simulink library "environment_lib"  (R2016b)
settings: Solver=ode45  StartTime=0.0  StopTime=10.0  RelTol=1e-3  EnableMultiTasking=on
undefined symbols (not defined in the file or in its folder): DT_aero, DT_grav, DT_solar, env_acc_eci, fsw_params, init_pos_eci, init_vel_eci, mag_vector_eci, MD_SC_resdipole, sun_vec_eci
libraries: time_conversion_lib x2, bus_stubs_template x2, GPS_time_lib x1, coord_rotation_lib x1, disturbances_lib x1, tle2eci_coarse_lib x1
settings Model: Creator=bbarz_000  LastModifiedBy=evich
settings DataIOCC: LimitDataPoints=on
settings OptimizationCC: LifeSpan=inf
settings DebuggingCC: AllowSymbolicDim=off  SFUnexpectedBacktrackingDiag=warning  SFNoUnconditionalDefaultTransitionDiag=warning  SFExecutionAtInitializationDiag=none
settings GRTTargetCC: TargetLangStandard=C89/C90 (ANSI)  GeneratePreprocessorConditionals=Disable all
settings ConfigComp: CovMetricSettings=dw  CovHtmlReporting=on  CovSaveCumulativeToWorkspaceVar=on  CovSaveSingleToWorkspaceVar=on  CovExternalEMLEnable=off

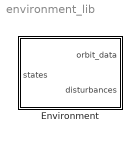
== system environment_lib ==
  Environment : Subsystem

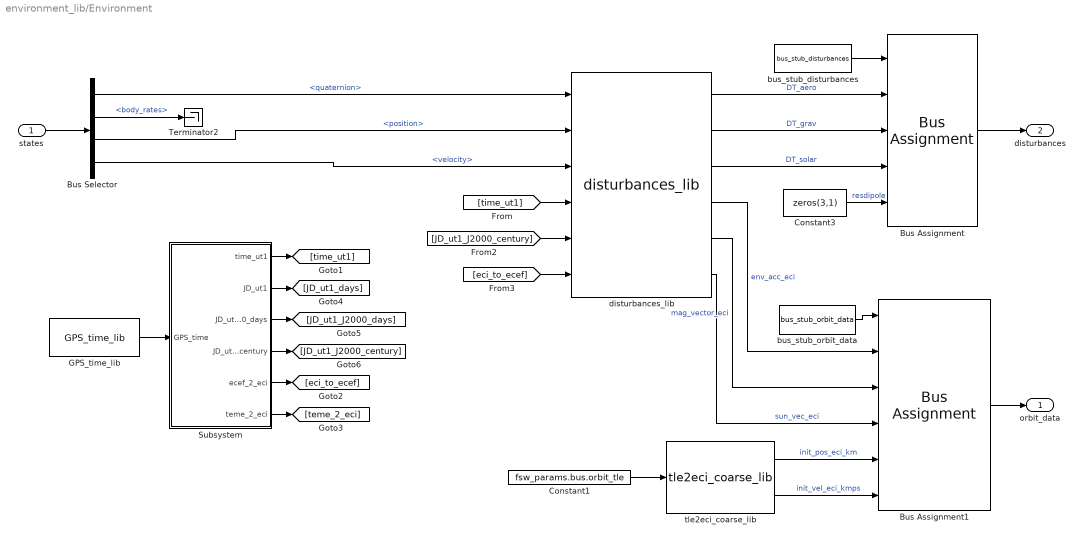
== system environment_lib/Environment ==
  states : Inport  OutDataTypeStr=Bus: states
  Bus Assignment : BusAssignment  AssignedSignals=DT_aero,DT_grav,DT_solar,MD_SC_resdipole
  Bus Assignment1 : BusAssignment  AssignedSignals=env_acc_eci,mag_vector_eci,sun_vec_eci,init_pos_eci,init_vel_eci
  Bus Selector : BusSelector  OutputSignals=quaternion,body_rates,position,velocity
  Constant1 : Constant  Value=fsw_params.bus.orbit_tle
  Constant3 : Constant  Value=zeros(3,1)
  GPS_time_lib : GPS_time_lib/GPS_time_lib
  Subsystem : Subsystem
  Terminator2 : Terminator
  bus_stub_disturbances : bus_stubs_template/bus_stub_disturbances
  bus_stub_orbit_data : bus_stubs_template/bus_stub_orbit_data
  disturbances_lib : disturbances_lib/disturbances_lib
  tle2eci_coarse_lib : tle2eci_coarse_lib/tle2eci_coarse_lib
  orbit_data : Outport
  disturbances : Outport  Port=2
  wires:
  tle2eci_coarse_lib/2 -> Bus Assignment1/6  "init_vel_eci_kmps"
  tle2eci_coarse_lib/1 -> Bus Assignment1/5  "init_pos_eci_km"
  Constant1/1 -> tle2eci_coarse_lib/1
  bus_stub_disturbances/1 -> Bus Assignment/1
  Bus Assignment/1 -> disturbances/1
  states/1 -> Bus Selector/1
  Bus Selector/1 -> disturbances_lib/1  "<quaternion>"
  Bus Selector/2 -> Terminator2/1  "<body_rates>"
  Bus Selector/3 -> disturbances_lib/2  "<position>"
  Bus Selector/4 -> disturbances_lib/3  "<velocity>"
  [time_ut1] -> disturbances_lib/4
  Constant3/1 -> Bus Assignment/5  "resdipole"
  bus_stub_orbit_data/1 -> Bus Assignment1/1
  Bus Assignment1/1 -> orbit_data/1
  disturbances_lib/6 -> Bus Assignment1/4  "sun_vec_eci"
  Subsystem/3(JD_ut1_J2000_days) -> [JD_ut1_J2000_days]
  Subsystem/1(time_ut1) -> [time_ut1]
  Subsystem/2(JD_ut1) -> [JD_ut1_days]
  Subsystem/4(JD_ut1_J2000_century) -> [JD_ut1_J2000_century]
  Subsystem/6(teme_2_eci) -> [teme_2_eci]
  Subsystem/5(ecef_2_eci) -> [eci_to_ecef]
  [JD_ut1_J2000_century] -> disturbances_lib/5
  [eci_to_ecef] -> disturbances_lib/6
  GPS_time_lib/1 -> Subsystem/1(GPS_time)
  disturbances_lib/1 -> Bus Assignment/2  "DT_aero"
  disturbances_lib/2 -> Bus Assignment/3  "DT_grav"
  disturbances_lib/3 -> Bus Assignment/4  "DT_solar"
  disturbances_lib/4 -> Bus Assignment1/2  "env_acc_eci"
  disturbances_lib/5 -> Bus Assignment1/3  "mag_vector_eci"

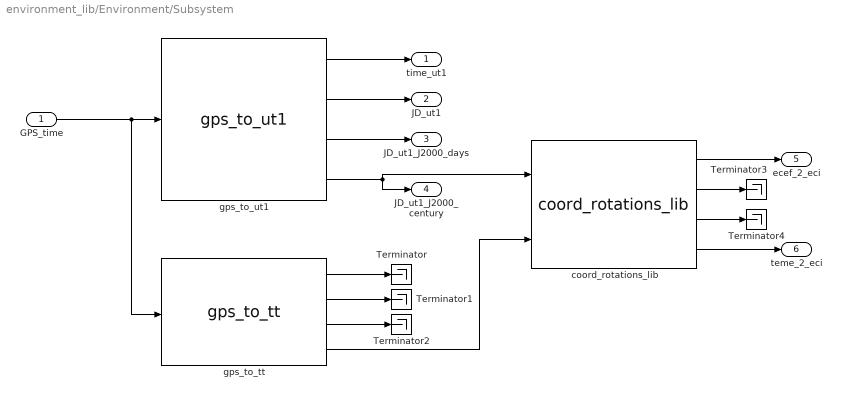
== system environment_lib/Environment/Subsystem ==
  GPS_time : Inport
  Terminator{,1..4} (5 alike) : Terminator
  coord_rotations_lib : coord_rotation_lib/coord_rotations_lib
  gps_to_tt : time_conversion_lib/gps_to_tt
  gps_to_ut1 : time_conversion_lib/gps_to_ut1
  time_ut1 : Outport
  JD_ut1 : Outport  Port=2
  JD_ut1_J2000_days : Outport  Port=3
  JD_ut1_J2000_century : Outport  Port=4
  ecef_2_eci : Outport  Port=5
  teme_2_eci : Outport  Port=6
  wires:
  GPS_time/1 -> gps_to_ut1/1, gps_to_tt/1
  gps_to_ut1/4 -> JD_ut1_J2000_century/1, coord_rotations_lib/1
  gps_to_tt/4 -> coord_rotations_lib/2
  gps_to_ut1/1 -> time_ut1/1
  gps_to_ut1/2 -> JD_ut1/1
  gps_to_ut1/3 -> JD_ut1_J2000_days/1
  gps_to_tt/1 -> Terminator/1
  gps_to_tt/3 -> Terminator2/1
  gps_to_tt/2 -> Terminator1/1
  coord_rotations_lib/2 -> Terminator3/1
  coord_rotations_lib/3 -> Terminator4/1
  coord_rotations_lib/1 -> ecef_2_eci/1
  coord_rotations_lib/4 -> teme_2_eci/1
